simulink model "if_grading_system"  (R2021a)
settings: Solver=FixedStepDiscrete  StartTime=0.0  StopTime=10.0  RelTol=1e-3  EnableMultiTasking=on
settings Model: Creator=omar  LastModifiedBy=omar
settings DataIOCC: ReturnWorkspaceOutputs=off
settings OptimizationCC: DefaultParameterBehavior=Inlined  InlineInvariantSignals=on  EnableMemcpy=off  LifeSpan=1  EfficientTunableParamExpr=on
settings DebuggingCC: UnderspecifiedInitializationDetection=Classic  MergeDetectMultiDrivingBlocksExec=none  SFMachineParentedDataDiag=warning  ArithmeticOperatorsInVariantConditions=warning
settings ModelReferenceCC: PropagateSignalLabelsOutOfModel=off
settings SFSimCC: MATLABDynamicMemAlloc=off  CustomCodeUndefinedFunction=UseInterfaceOnly
settings RTWCC: SystemTargetFile=ert.tlc  GenCodeOnly=on  TemplateMakefile=ert_default_tmf  GenerateReport=on  IncludeHyperlinkInReport=on  LaunchReport=on  GenerateTraceInfo=on  GenerateTraceReport=on  GenerateTraceReportSl=on  GenerateTraceReportSf=on  GenerateTraceReportEml=on
settings CodeAppCC: ForceParamTrailComments=on  IgnoreCustomStorageClasses=off  OperatorAnnotations=on  SimulinkDataObjDesc=on  SFDataObjDesc=on  MATLABFcnDesc=on  InsertBlockDesc=on  StateflowObjectComments=on  MATLABSourceComments=on
settings ERTTargetCC: MultiwordLength=2048  GenerateSampleERTMain=on  InlinedParameterPlacement=NonHierarchical  ERTCustomFileTemplate=example_file_process.tlc

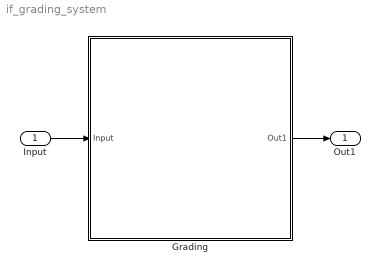
== system if_grading_system ==
  Input : Inport
  Grading : Subsystem
  Out1 : Outport
  wires:
  Input/1 -> Grading/1(Input)
  Grading/1(Out1) -> Out1/1

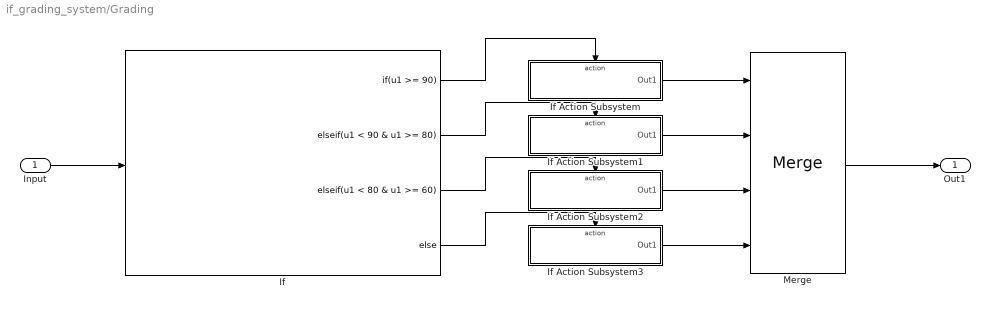
== system if_grading_system/Grading ==
  Input : Inport
  If : If  IfExpression=u1 >= 90  ElseIfExpressions=u1 < 90 & u1 >= 80,u1 < 80 & u1 >= 60
  If Action Subsystem : Subsystem  TreatAsAtomicUnit=on
  If Action Subsystem1 : Subsystem  TreatAsAtomicUnit=on
  If Action Subsystem2 : Subsystem  TreatAsAtomicUnit=on
  If Action Subsystem3 : Subsystem  TreatAsAtomicUnit=on
  Merge : Merge  Inputs=4
  Out1 : Outport
  wires:
  If Action Subsystem2/1(Out1) -> Merge/3
  If/1 -> If Action Subsystem/Action
  If Action Subsystem3/1(Out1) -> Merge/4
  If/4 -> If Action Subsystem3/Action
  If/2 -> If Action Subsystem1/Action
  Input/1 -> If/1
  If Action Subsystem1/1(Out1) -> Merge/2
  If/3 -> If Action Subsystem2/Action
  Merge/1 -> Out1/1
  If Action Subsystem/1(Out1) -> Merge/1

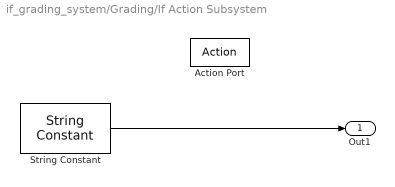
== system if_grading_system/Grading/If Action Subsystem ==
  Action Port : ActionPort  ActionPortLabel=if(u1 >= 90)
  String Constant : StringConstant  String="\"Excellent\""
  Out1 : Outport
  wires:
  String Constant/1 -> Out1/1

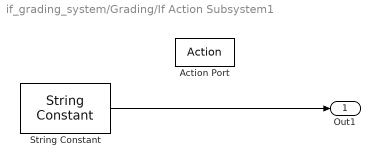
== system if_grading_system/Grading/If Action Subsystem1 ==
  Action Port : ActionPort  ActionPortLabel=elseif(u1 < 90 & u1 >= 80)
  String Constant : StringConstant  String="\"Very Good\""
  Out1 : Outport
  wires:
  String Constant/1 -> Out1/1

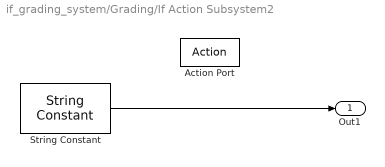
== system if_grading_system/Grading/If Action Subsystem2 ==
  Action Port : ActionPort  ActionPortLabel=elseif(u1 < 80 & u1 >= 60)
  String Constant : StringConstant  String="\"Pass\""
  Out1 : Outport
  wires:
  String Constant/1 -> Out1/1

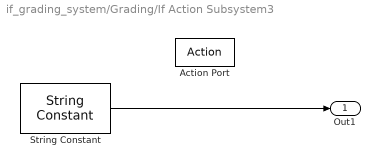
== system if_grading_system/Grading/If Action Subsystem3 ==
  Action Port : ActionPort  ActionPortLabel=else
  String Constant : StringConstant  String="\"Fail\""
  Out1 : Outport
  wires:
  String Constant/1 -> Out1/1
